simulink model "Schnittstellendummy_Gewerk1"  (R2015b)
settings: Solver=VariableStepAuto  StartTime=0.0  StopTime=1000.0  RelTol=1e-3
libraries: simulink x2
settings Model: Creator=atlabor  LastModifiedBy=atlabor

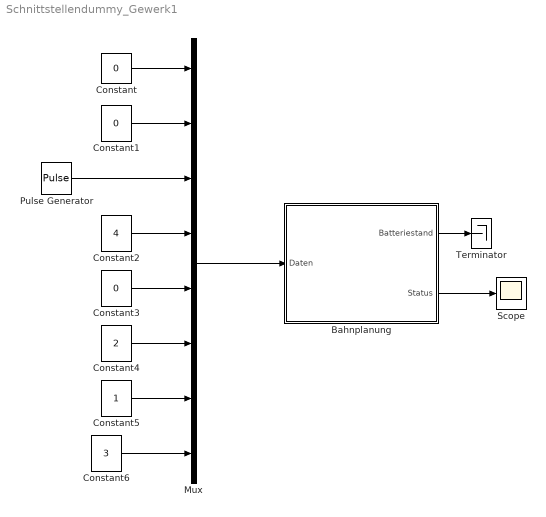
== system Schnittstellendummy_Gewerk1 ==
  Bahnplanung : Subsystem
  Constant : Constant  Value=0
  Constant1 : Constant  Value=0
  Constant2 : Constant  Value=4  OutDataTypeStr=double
  Constant3 : Constant  Value=0  OutDataTypeStr=double
  Constant4 : Constant  Value=2  OutDataTypeStr=double
  Constant5 : Constant  OutDataTypeStr=double
  Constant6 : Constant  Value=3  OutDataTypeStr=double
  Mux : Mux  Inputs=8
  Pulse Generator : DiscretePulseGenerator  PulseType=Time based  Period=100  PulseWidth=50
  Scope : Scope
  Terminator : Terminator
  wires:
  Bahnplanung/1(Batteriestand) -> Terminator/1
  Mux/1 -> Bahnplanung/1(Daten)
  Bahnplanung/2(Status) -> Scope/1
  Constant/1 -> Mux/1
  Constant1/1 -> Mux/2
  Pulse Generator/1 -> Mux/3
  Constant2/1 -> Mux/4
  Constant3/1 -> Mux/5
  Constant4/1 -> Mux/6
  Constant5/1 -> Mux/7
  Constant6/1 -> Mux/8

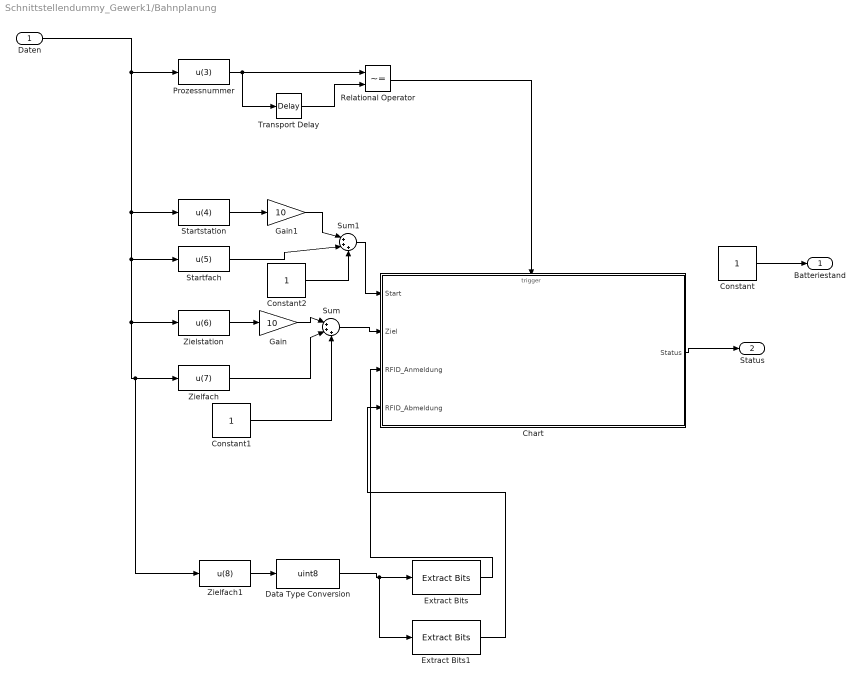
== system Schnittstellendummy_Gewerk1/Bahnplanung ==
  Daten : Inport
  Chart : Stateflow chart  TreatAsAtomicUnit=on
  Constant : Constant
  Constant1 : Constant
  Constant2 : Constant
  Data Type Conversion : DataTypeConversion  OutDataTypeStr=uint8
  Extract Bits : simulink/Logic and Bit Operations/Extract Bits  bitsToExtract=Range of bits  numBits=8  bitIdxRange=[0]  outScalingMode=Treat bit field as an integer
  Extract Bits1 : simulink/Logic and Bit Operations/Extract Bits  bitsToExtract=Range of bits  numBits=8  bitIdxRange=[1]  outScalingMode=Treat bit field as an integer
  Gain : Gain  Gain=10
  Gain1 : Gain  Gain=10
  Prozessnummer : Fcn  Expr=u(3)
  Relational Operator : RelationalOperator  Operator=~=  OutDataTypeStr=boolean
  Startfach : Fcn  Expr=u(5)
  Startstation : Fcn  Expr=u(4)
  Sum : Sum  Inputs=|+++
  Sum1 : Sum  Inputs=|+++
  Transport Delay : TransportDelay  DelayTime=2
  Zielfach : Fcn  Expr=u(7)
  Zielfach1 : Fcn  Expr=u(8)
  Zielstation : Fcn  Expr=u(6)
  Batteriestand : Outport
  Status : Outport  Port=2
  wires:
  Constant/1 -> Batteriestand/1
  Chart/1(Status) -> Status/1
  Daten/1 -> Prozessnummer/1, Zielfach1/1, Zielfach/1, Zielstation/1, Startfach/1, Startstation/1
  Zielstation/1 -> Gain/1
  Gain/1 -> Sum/1
  Zielfach/1 -> Sum/2
  Sum/1 -> Chart/2(Ziel)
  Constant1/1 -> Sum/3
  Startstation/1 -> Gain1/1
  Gain1/1 -> Sum1/1
  Startfach/1 -> Sum1/2
  Sum1/1 -> Chart/1(Start)
  Constant2/1 -> Sum1/3
  Relational Operator/1 -> Chart/Trigger
  Transport Delay/1 -> Relational Operator/2
  Prozessnummer/1 -> Transport Delay/1, Relational Operator/1
  Zielfach1/1 -> Data Type Conversion/1
  Data Type Conversion/1 -> Extract Bits1/1, Extract Bits/1
  Extract Bits1/1 -> Chart/4(RFID_Abmeldung)
  Extract Bits/1 -> Chart/3(RFID_Anmeldung)

== stateflow chart Schnittstellendummy_Gewerk1/Bahnplanung/Chart ==
  state Bahnplanung
    state Warten
      entry:Status=0;
    state Auftragerhalten
      entry:Status=1;
    state Start_erreicht
    state Ziel_erreicht
      entry:Status=1;
    state Werkstueck_beim_RFID
      entry:Status=3;
    state Werkstueck_befoerdern
      entry:Status=1;
    state Werkstueck_beim_RFID2
      entry:Status=2;
    (default) -> Warten
    Auftragerhalten -> Start_erreicht : after(20,sec)
    Warten -> Auftragerhalten : Neuer_Auftrag
    Ziel_erreicht -> Warten : after(5,sec)
    Start_erreicht -> Werkstueck_beim_RFID : after(5,sec)
    Werkstueck_beim_RFID2 -> Ziel_erreicht : [RFID_Anmeldung==1]
    Werkstueck_beim_RFID -> Werkstueck_befoerdern : [RFID_Abmeldung==1]
    Werkstueck_befoerdern -> Werkstueck_beim_RFID2 : after(10,sec)
  data: Status output; Start input; Ziel input; RFID_Anmeldung input; RFID_Abmeldung input
  events: Neuer_Auftrag input RISING_EDGE_EVENT
